simulink model "single_track_sim"  (R2024a)
settings: Solver=VariableStepAuto  StartTime=0.0  StopTime=100  RelTol=1e-3
undefined symbols (not defined in the file or in its folder): DiscIntNeverNeededParam
libraries: simulink x3, autolibshared x1
settings Model: Creator=pair-andres  LastModifiedBy=pair-andres

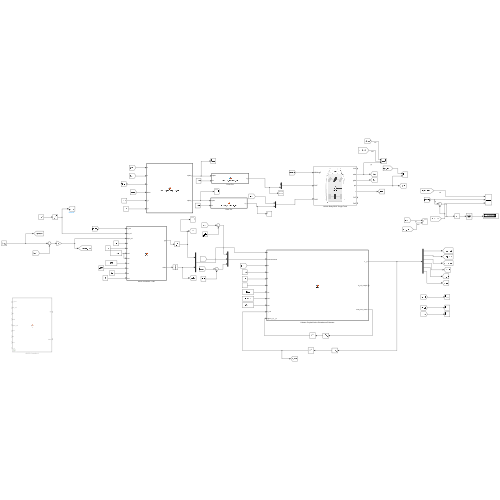
[thumbnail: Simulink's stored preview of the top-level diagram]
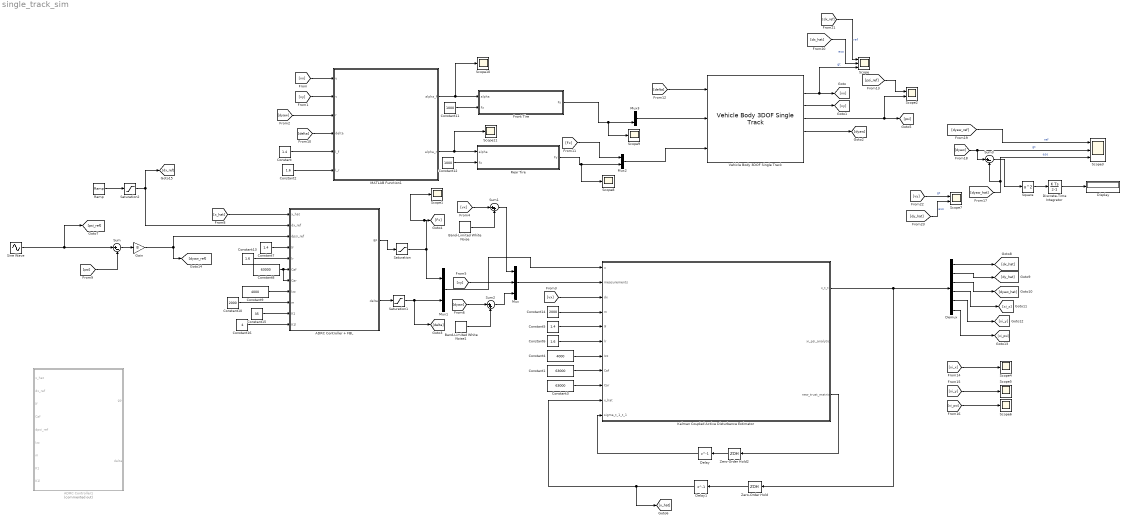
== system single_track_sim ==
  ADRC Controller + FBL : MATLAB Function  TreatAsAtomicUnit=on
  ADRC Controller1 : MATLAB Function  Commented=on  TreatAsAtomicUnit=on
  Band-Limited White Noise : simulink/Sources/Band-Limited White Noise  Cov=[0.001]  Ts=0.1  seed=[23341]
  Band-Limited White Noise1 : simulink/Sources/Band-Limited White Noise  Cov=[0.0000001]  Ts=0.05  seed=[23341]
  Constant : Constant  Value=1.4
  Constant1 : Constant  Value=63000
  Constant10 : Constant  Value=2000
  Constant11 : Constant  Value=1000
  Constant12 : Constant  Value=1000
  Constant13 : Constant  Value=1.6
  Constant14 : Constant  Value=2000
  Constant15 : Constant  Value=35
  Constant16 : Constant  Value=4
  Constant2 : Constant  Value=1.6
  Constant3 : Constant  Value=63000
  Constant4 : Constant  Value=4000
  Constant5 : Constant  Value=1.4
  Constant6 : Constant  Value=1.6
  Constant7 : Constant  Value=1.4
  Constant8 : Constant  Value=63000
  Constant9 : Constant  Value=4000
  Delay : Delay  DelayLength=1  SampleTime=0.01
  Delay1 : Delay  DelayLength=1  SampleTime=0.01
  Demux : Demux  Outputs=6
  Discrete-Time Integrator : DiscreteIntegrator  SampleTime=0.01  ICPrevOutput=DiscIntNeverNeededParam  ICPrevScaledInput=DiscIntNeverNeededParam
  Display : Display
  Front Tire : MATLAB Function  TreatAsAtomicUnit=on
  Gain : Gain  Gain=8
  Kalman Coupled Active Disturbance Estimator : MATLAB Function  TreatAsAtomicUnit=on
  MATLAB Function1 : MATLAB Function  TreatAsAtomicUnit=on
  Mux : Mux  Inputs=3
  Mux1 : Mux  Inputs=2
  Mux2 : Mux  Inputs=2
  Mux3 : Mux  Inputs=2
  Ramp : simulink/Sources/Ramp  slope=0.03  start=5  InitialOutput=10
  Rear Tire : MATLAB Function  TreatAsAtomicUnit=on
  Saturation : Saturate  UpperLimit=2000  LowerLimit=-2000
  Saturation1 : Saturate  UpperLimit=0.262  LowerLimit=-0.262
  Saturation2 : Saturate  UpperLimit=50
  Scope : Scope  NumInputPorts=3
  Scope{1,4..6,8..11} (8 alike) : Scope
  Scope2 : Scope  NumInputPorts=2
  Scope3 : Scope  NumInputPorts=3
  Scope7 : Scope  NumInputPorts=2
  Sine Wave : Sin  Amplitude=0.3  Frequency=0.1  SampleTime=0
  Square : Math  Operator=square
  Sum : Sum  Inputs=|+-
  Sum1 : Sum  Inputs=|++
  Sum2 : Sum  Inputs=|++
  Sum3 : Sum  Inputs=|+-
  Vehicle Body 3DOF Single Track : autolibshared/Vehicle Body 3DOF Single Track  trackMode=Single (bicycle)  inputMode=External forces  frontSteerMode=on  rearSteerMode=off  windMode=off  muMode=off  extFMode=off  extMMode=off  htchFMode=off  htchMMode=off  extXo=off  extpsio=off  extxdoto=off  extro=off  extYo=off  extTamb=off  extydoto=off  aMode=2  NF=2  NR=2  m=2000  a=1.4  b=1.6  h=0.35  dh=1  hh=0.2  X_o=0  xdot_o=5  CalphaMode=off  sigmaMode=on  d=0  hl=0  w=[1.4,1.4]  Cy_f=12e3  Cy_r=11e3  sigma_f=.1  sigma_r=.1  alpha_f_brk=[-.1 .1]  Cy_f_data=[-9e3 9e3]  alpha_r_brk=[-.1 .1]  Cy_r_data=[-9e3 9e3]  Y_o=0  ydot_o=0  Izz=4000  psi_o=0  r_o=0  Af=2  Cd=.3  Cl=.1  Cpm=.1  beta_w=[0 0.01:0.01:0.3]  Cs=[0 0.01:0.01:0.3]  Cym=[0 1e-6:0.01:0.3]  Pabs=101325  Tair=273  g=9.81  mu=1  xdot_tol=.01  Fznom=5000  Fxtire_sat=7e4  Fytire_sat=7e4  longOff=0  latOff=0  vertOff=0  wrapAng=off
  Zero-Order Hold : ZeroOrderHold  SampleTime=0.01
  Zero-Order Hold2 : ZeroOrderHold  SampleTime=0.01
  wires:
  Constant/1 -> MATLAB Function1/5(l_f)
  Constant2/1 -> MATLAB Function1/6(l_r)
  Vehicle Body 3DOF Single Track/2 -> Scope/3, [vx]  "gt"
  Vehicle Body 3DOF Single Track/3 -> [vy]
  [vx] -> MATLAB Function1/1(u)
  [vy] -> MATLAB Function1/2(v)
  Vehicle Body 3DOF Single Track/5 -> [dyaw]
  [dyaw] -> MATLAB Function1/3(r)
  MATLAB Function1/1(alpha_f) -> Scope10/1, Front Tire/1(alpha)
  MATLAB Function1/2(alpha_r) -> Scope11/1, Rear Tire/1(alpha)
  Constant1/1 -> Kalman Coupled Active Disturbance Estimator/8(Caf)
  Constant3/1 -> Kalman Coupled Active Disturbance Estimator/9(Car)
  Constant4/1 -> Kalman Coupled Active Disturbance Estimator/7(Izz)
  Constant6/1 -> Kalman Coupled Active Disturbance Estimator/6(lr)
  Constant5/1 -> Kalman Coupled Active Disturbance Estimator/5(lf)
  Constant14/1 -> Kalman Coupled Active Disturbance Estimator/4(m)
  [vx] -> Kalman Coupled Active Disturbance Estimator/3(dx)
  [vy] -> Mux/2
  Mux/1 -> Kalman Coupled Active Disturbance Estimator/2(measurements)
  Constant7/1 -> ADRC Controller + FBL/4(lf)
  Constant8/1 -> ADRC Controller + FBL/7(Car), ADRC Controller + FBL/6(Caf)
  Sine Wave/1 -> [psi_ref], Sum/1
  [psi] -> Sum/2
  Sum/1 -> Gain/1
  Gain/1 -> ADRC Controller + FBL/3(dpsi_ref), [dyaw_ref]
  Zero-Order Hold/1 -> Delay1/1
  Kalman Coupled Active Disturbance Estimator/1(x_t_t) -> Demux/1, Zero-Order Hold/1
  Delay1/1 -> [x_hat], Kalman Coupled Active Disturbance Estimator/10(x_hat)
  Zero-Order Hold2/1 -> Delay/1
  Kalman Coupled Active Disturbance Estimator/3(new_trust_matrix) -> Zero-Order Hold2/1
  Delay/1 -> Kalman Coupled Active Disturbance Estimator/11(sigma_t_1_t_1)
  [x_hat] -> ADRC Controller + FBL/1(x_hat)
  ADRC Controller + FBL/1(gp) -> Saturation/1
  ADRC Controller + FBL/2(delta) -> Saturation1/1
  Mux1/1 -> Kalman Coupled Active Disturbance Estimator/1(u)
  Saturation/1 -> Mux1/1, Scope1/1, [Fx]
  Saturation1/1 -> [delta], Mux1/2
  [delta] -> MATLAB Function1/4(delta)
  Constant11/1 -> Front Tire/2(Fz)
  Constant12/1 -> Rear Tire/2(Fz)
  [Fx] -> Mux2/1
  Rear Tire/1(Fy) -> Scope8/1, Mux2/2
  Mux2/1 -> Vehicle Body 3DOF Single Track/3
  Front Tire/1(Fy) -> Scope9/1, Mux3/2
  Mux3/1 -> Vehicle Body 3DOF Single Track/2
  [delta] -> Vehicle Body 3DOF Single Track/1
  Vehicle Body 3DOF Single Track/4 -> Scope2/2, [psi]
  Saturation2/1 -> ADRC Controller + FBL/2(dx_ref), [dx_ref]
  [psi_ref] -> Scope2/1
  Demux/1 -> [dx_hat]
  Demux/2 -> [dy_hat]
  Demux/3 -> [dyaw_hat]
  Demux/4 -> [xi_x]
  Demux/5 -> [xi_y]
  Demux/6 -> [xi_psi]
  [dyaw_ref] -> Scope3/1  "ref"
  [dyaw] -> Scope3/2, Sum3/1  "gt"
  [dyaw_hat] -> Sum3/2, Scope3/3  "eso"
  [xi_x] -> Scope4/1
  [xi_y] -> Scope5/1
  [xi_psi] -> Scope6/1
  [dx_hat] -> Scope/2  "eso"
  [dx_ref] -> Scope/1  "ref"
  [vy] -> Scope7/1  "gt"
  [dy_hat] -> Scope7/2  "eso"
  Constant15/1 -> ADRC Controller + FBL/10(K1)
  Constant16/1 -> ADRC Controller + FBL/11(K1l)
  Ramp/1 -> Saturation2/1
  [vx] -> Sum1/1
  Band-Limited White Noise/1 -> Sum1/2
  Sum1/1 -> Mux/1
  [dyaw] -> Sum2/1
  Band-Limited White Noise1/1 -> Sum2/2
  Sum2/1 -> Mux/3
  Square/1 -> Discrete-Time Integrator/1
  Sum3/1 -> Square/1
  Discrete-Time Integrator/1 -> Display/1
  Constant13/1 -> ADRC Controller + FBL/5(lr)
  Constant9/1 -> ADRC Controller + FBL/8(Izz)
  Constant10/1 -> ADRC Controller + FBL/9(m)

== matlab function single_track_sim/MATLAB Function1 ==
  data: u input; alpha_f output; v input; r input; delta input; l_f input; l_r input; alpha_r output
function [alpha_f, alpha_r] = calc_bicycle_slip_angles(u, v, r, delta, l_f, l_r)
%#codegen
% Calculates the front and rear slip angles for a single-track (bicycle) model.
%
% INPUTS:
%   u:        Vehicle longitudinal velocity (at CG) [m/s]
%   v:        Vehicle lateral velocity (at CG) [m/s]
%   r:        Vehicle yaw rate [rad/s]
%   delta:    Front steering angle (from controller) [rad]
%   l_f:      Distance from CG to front axle [m]
%   l_r:      Distance from CG to rear axle [m]
%
% OUTPUTS:
%   alpha_f:  Front axle slip angle [rad]
%   alpha_r:  Rear axle slip angle [rad]

% --- 1. Calculate velocity angle at the front axle ---
% We find the lateral and longitudinal velocity components at the point
% of the front axle (on the vehicle centerline).
% v_y = v (at CG) + r * l_f (tangential velocity from yaw)
% v_x = u (at CG), since y=0, there is no component from yaw
theta_v_f = atan2(v + r * l_f, u);

% --- 2. Calculate velocity angle at the rear axle ---
% We find the velocity components at the point of the rear axle.
% v_y = v (at CG) - r * l_r (tangential velocity from yaw)
theta_v_r = atan2(v - r * l_r, u);

% --- 3. Calculate Slip Angles ---
% Slip angle is the difference between where the wheel is
% pointing (delta) and where the wheel is going (theta_v).

% Front: Steer angle is delta, velocity angle is theta_v_f
alpha_f = delta - theta_v_f;

% Rear: Steer angle is 0, velocity angle is theta_v_r
alpha_r = 0 - theta_v_r;

end

== matlab function single_track_sim/Rear Tire ==
  data: alpha input; Fy output; Fz input
function Fy = simple_pacejka_lat(alpha, Fz)

    % Implements the simple Pacejka '89 lateral force model.
    %
    % INPUTS:
    %   alpha:  Tire Slip Angle (radians)
    %   Fz:     Vertical Load on the tire (Newtons)
    %
    % OUTPUT:
    %   Fy:     Lateral Force (Newtons)
    
    % TIRE PACEJKA PARAMS:
    %   B:      Stiffness Factor
    %   C:      Shape Factor
    %   D:      Peak Factor (Peak friction coefficient, mu_y)
    %   E:      Curvature Factor
    
    B = 22; C = 1.8; D=1.6; E = 0.8;
    
    % --- Safety Check: Ensure Fz is positive ---
    % The formula assumes positive vertical load.
    Fz_pos = max(0, Fz);
    
    % --- 1. Calculate Peak Lateral Force ---
    % D is the friction coefficient, so F_peak = D * Fz
    F_peak = D * Fz_pos;
    
    % --- 2. Composite Slip Term ---
    % This is the main input to the sine function
    x = B * alpha;
    
    % --- 3. Pacejka '89 "Magic Formula" ---
    % This is the core equation
    Fy = F_peak * sin(C * atan(x - E * (x - atan(x))));

end

== matlab function single_track_sim/Front Tire ==
  data: alpha input; Fy output; Fz input
function Fy = simple_pacejka_lat(alpha, Fz)

    % Implements the simple Pacejka '89 lateral force model.
    %
    % INPUTS:
    %   alpha:  Tire Slip Angle (radians)
    %   Fz:     Vertical Load on the tire (Newtons)
    %
    % OUTPUT:
    %   Fy:     Lateral Force (Newtons)
    
    % TIRE PACEJKA PARAMS:
    %   B:      Stiffness Factor
    %   C:      Shape Factor
    %   D:      Peak Factor (Peak friction coefficient, mu_y)
    %   E:      Curvature Factor
    
    B = 22; C = 1.8; D=1.6; E = 0.8;
    
    % --- Safety Check: Ensure Fz is positive ---
    % The formula assumes positive vertical load.
    Fz_pos = max(0, Fz);
    
    % --- 1. Calculate Peak Lateral Force ---
    % D is the friction coefficient, so F_peak = D * Fz
    F_peak = D * Fz_pos;
    
    % --- 2. Composite Slip Term ---
    % This is the main input to the sine function
    x = B * alpha;
    
    % --- 3. Pacejka '89 "Magic Formula" ---
    % This is the core equation
    Fy = F_peak * sin(C * atan(x - E * (x - atan(x))));

end

== matlab function single_track_sim/ADRC Controller + FBL ==
  data: gp output; x_hat input; dx_ref input; dpsi_ref input; lf input; delta output size=[1]; lr input; Caf input; Car input; Izz input; m input; K1 input; K1l input
function [gp, delta] = fcn(x_hat, dx_ref, dpsi_ref, lf, lr, Caf, Car, Izz, m, K1, K1l)
% Implements a model-based ADRC controller by actively canceling
% the known linear vehicle dynamics and the estimated disturbance.

% --- 1. Unpack State Vector ---
% We assume the state vector is: x_hat = [vx, vy, r, xi_x, xi_y, xi_psi]'
dx   = x_hat(1); % vx (forward velocity)
dy   = x_hat(2); % vy (lateral velocity)
dpsi = x_hat(3); % r  (yaw rate)
xi_hat_x   = x_hat(4); % Estimated x-disturbance
xi_hat_y   = x_hat(5); % Estimated y-disturbance
xi_hat_psi = x_hat(6); % Estimated psi-disturbance

% --- 2. Longitudinal Control (gp) ---
% Model: m*dvx = gp + xi_x
% This controller cancels the disturbance and applies a P-controller
% on velocity error.
U0_x = K1l*(dx_ref - dx) - (xi_hat_x / m);
gp = m * U0_x;

% --- 3. Lateral/Yaw Control (delta) ---
% This is the new, model-based ADRC.

% 3.1. Calculate linear coupling terms (Nv, Nr)
% These are the terms from your 'A_aug' matrix that couple vy and r.
% (We add a small epsilon to dx to avoid division by zero if the car stops)
vx = dx + 1e-6; 
Nv = -(2*Caf*lf - 2*Car*lr) / (Izz * vx);
Nr = -(2*Caf*lf^2 + 2*Car*lr^2) / (Izz * vx);

% 3.2. Define the "virtual control" (U0_psi)
% This is the total yaw acceleration we want to command.
% U0_psi = (Reference Accel) + (PD Control) - (Linear Feedback) - (Disturbance Feedback)

psi_ddot_ref = 0; % Assuming reference yaw acceleration is 0 for path following

linear_feedback = (Nv * dy + Nr * dpsi);
disturbance_feedback = (xi_hat_psi / Izz);
pd_control = K1*(dpsi_ref - dpsi); % Your P-controller on rate error

U0_psi = psi_ddot_ref + pd_control - linear_feedback - disturbance_feedback;

% 3.3. Invert the linear control model (B_lin) to find delta
% Our linear model's control input part is: ddot_psi = ... + (2*Caf*lf / Izz) * delta
% We set U0_psi equal to this known control part and solve for delta.
B_lin_psi = (2*Caf*lf) / Izz;
delta = U0_psi / B_lin_psi;

% (Optional) Add saturation to the steering angle
% max_steer = 0.4; % radians
% delta = max(min(delta, max_steer), -max_steer);

end

== matlab function single_track_sim/ADRC Controller1 ==
  data: gp output; x_hat input; delta output size=[1]; dx_ref input; lf input; Caf input; dpsi_ref input; Izz input; m input; K1 input; K1l input
function [gp, delta] = fcn(x_hat, dx_ref, lf, Caf, dpsi_ref, Izz,  m, K1, K1l)


% dx = x_hat(1)
dx = x_hat(1);
dy = x_hat(2);
dpsi = x_hat(3);
xi_hat_x = x_hat(3);
xi_hat_y = x_hat(5);
xi_hat_psi = x_hat(6); 

% ADRC Control Law:
delta = (Izz/(2*Caf*lf)) * (-xi_hat_psi/Izz - 0 + K1*(dpsi_ref - dpsi));
gp = (m) * (-xi_hat_x - 0 + K1l*(dx_ref - dx));
% delta = ((dx + dy + dpsi*lf)*Izz / (2*lf*Caf*max(1,dx))) * (-xi_hat_ddpsi + 0 - K1*(dpsi - dpsi_ref) - K2*(psi - psi_ref));

== matlab function single_track_sim/Kalman Coupled Active Disturbance Estimator ==
  data: u input; x_t_t output; measurements input; dx input; m input; lf input; lr input; Izz input; Caf input; Car input; x_hat input; sigma_t_1_t_1 input; xi_psi_analytic output; new_trust_matrix output
function [x_t_t, xi_psi_analytic, new_trust_matrix]= fcn(u, measurements, dx, m, lf, lr, Izz, Caf, Car, x_hat, sigma_t_1_t_1)

sigma_y_given_x = eye(3)*0.2; % 4 states in the measurements vector
sigma_x = eye(6)*0.01;

% Retrieve dy, dz from measurements
dy = measurements(2);
dpsi = measurements(3);

T = 0.01; % seconds

% A_aug = [
%     0, 0, 0, 1/m, 0, 0;
%     0, 0, 0, 0, 1/m, 0;
%     0, 0, 0, 0, 0, 1/Izz;
%     0, 0, 0, 0, 0, 0;
%     0, 0, 0, 0, 0, 0;
%     0, 0, 0, 0, 0, 0;
% ];

vx = dx;


% Linear Bicycle Model Terms
Yv = -(2*Caf + 2*Car) / (m * vx);
Yr = -vx - (2*Caf*lf - 2*Car*lr) / (m * vx);
Nv = -(2*Caf*lf - 2*Car*lr) / (Izz * vx);
Nr = -(2*Caf*lf^2 + 2*Car*lr^2) / (Izz * vx);

% Build the new, physically-correct A_aug matrix
% We assume vx dynamics are separate (e.g., dvx = 1/m * Fx_input + 1/m * xi_x)
A_aug = [
    0,   0,   0,   1/m,   0,     0;     % dvx equation (no coupling)
    0,   Yv,  Yr,  0,     1/m,   0;     % dvy equation (COUPLED)
    0,   Nv,  Nr,  0,     0,     1/Izz; % dr equation (COUPLED)
    0,   0,   0,   0,     0,     0;     % d(xi_x)
    0,   0,   0,   0,     0,     0;     % d(xi_y)
    0,   0,   0,   0,     0,     0      % d(xi_psi)
];

C_aug = [
   eye(3), zeros(3);
];




% Build matrix B which depends on state variables and complicated terms:

% b21 = 0;
% b22 = (1/m) * (2*Caf*dx/(dx+dy+dpsi*lf));
% 
% b41 = 0;
% b42 = (1/Izz) * (2*lf*Caf*dx/(dx+dy+dpsi*lf));

B_aug = [
    1/m, 0;
    0, 2*Caf/m;
    0, 2*Caf*lf/Izz;
    0, 0;
    0, 0;
    0, 0
];

% Discretize state-space with Zero Order Hold (ZOH):
Ad = eye(6) + A_aug*T;
Bd = T*B_aug;
Cd = C_aug;

% disp('vx')
% disp(dx)


% Predict (Time Update):
x_t_t_1 = Ad*x_hat + Bd*u;
sigma_t_t_1 = Ad * sigma_t_1_t_1 * Ad' + sigma_x;


% Update (Measurement Update):
Kt = sigma_t_t_1 * C_aug' * inv(C_aug*sigma_t_t_1*C_aug' + sigma_y_given_x);
x_t_t = x_t_t_1 + Kt * (measurements - C_aug*x_t_t_1);
sigma_t_t = sigma_t_t_1 - Kt * C_aug * sigma_t_t_1;

new_trust_matrix = sigma_t_t;



% Cobs = eye(6);
% Dobs = zeros(6,2);

% Build disturbance can we?
xi_psi_analytic = (-(2*lf*Caf*(dy+dpsi*lf)*cos(u(2)))/(dx+dy+dpsi*lf) + (2*lr*Car*(dy-dpsi*lf))/(dx) ) *(1/Izz);
